simulink model "GIL11_free_mechanism"  (R2019b)
settings: Solver=VariableStepAuto  StartTime=0.133  StopTime=1.0823  MaxStep=0.01  RelTol=1e-3
PreLoadFcn:
  | kinData_max = 0;
  | kinData_min = 0;
libraries: simulink x3
settings Model: Creator=admin-local  LastModifiedBy=admin-local

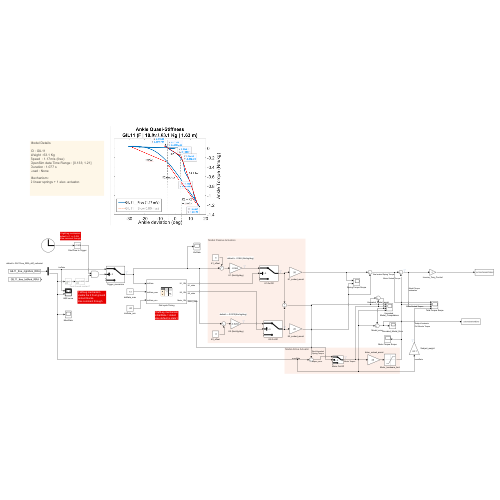
[thumbnail: Simulink's stored preview of the top-level diagram]
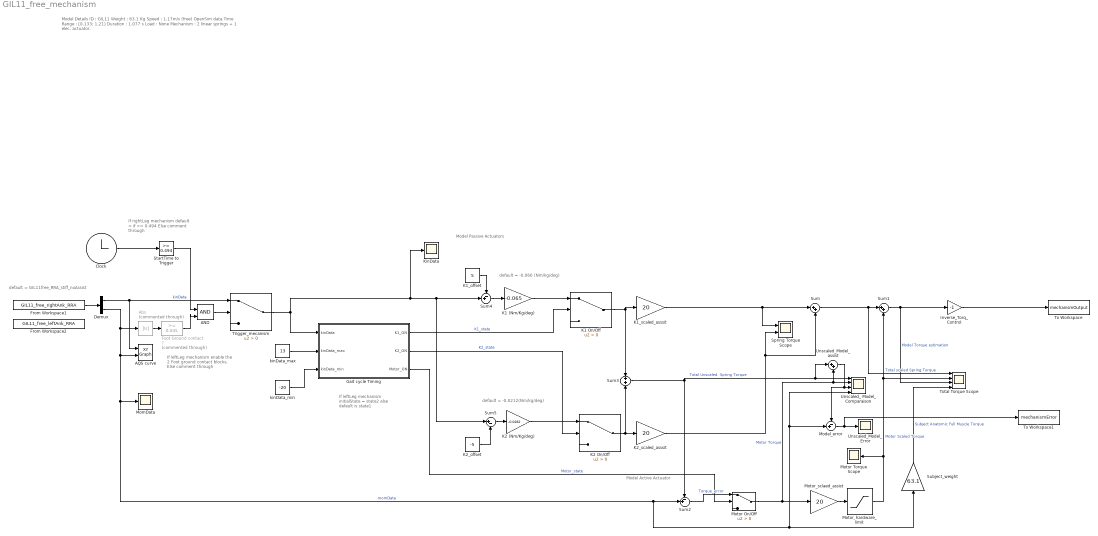
== system GIL11_free_mechanism ==
  note: Model Passive Actuators
  note: default = -0.066 (Nm/kg/deg)
  note: default = -0.0212(Nm/kg/deg)
  note: Model Active Actuator
  note: default = GIL11free_RRA_stiff_noAssist
  note: Model Details
      |
      | ID : GIL11
      | Weight : 63.1 Kg
      | Speed  : 1.17m/s (free)
      | OpenSim data Time Range : [0.133; 1.21]
      | Duration : 1.077 s
      | Load : None
      |
      | Mechanism :
      | 2 linear springs + 1 elec. actuator.
  note: If leftLeg mechanism
      | initialState = state2
      | else default is state1
  note: If rightLeg mechanism
      | default = if  >= 0.494
      | Else comment through
  note: If leftLeg mechanism
      | enable the 2 Foot ground contact blocks.
      | Else comment through
  AND : Logic  IconShape=distinctive  AllPortsSameDT=off  OutDataTypeStr=boolean
  AQS curve : simulink/Sinks/XY Graph  xmin=-1  xmax=1  ymin=-1  ymax=1  st=-1
  Abs : Abs  Commented=through
  Clock : Clock
  Demux : Demux  Outputs=2
  Foot Ground contact ? : simulink/Logic and Bit Operations/Compare To Constant  Commented=through  relop=>=  const=0.045  OutDataTypeStr=boolean
  From Workspace1 : FromWorkspace  VariableName=GIL11_free_rightAnk_RRA  OutputAfterFinalValue=Holding final value
  From Workspace2 : FromWorkspace  VariableName=GIL11_free_leftAnk_RRA  OutputAfterFinalValue=Holding final value
  Gait cycle Timing : State Transition Table  TreatAsAtomicUnit=on
  Inverse_Torq_Control : Gain  Gain=-1
  K1 (Nm/Kg/deg) : Gain  Gain=-0.065
  K1 On/Off : Switch  Criteria=u2 > Threshold
  "K1_offset " : Constant  Value=5
  K1_scaled_asssit : Gain  Gain=20
  K2 (Nm/Kg/deg) : Gain  Gain=-0.0282
  K2 On/Off : Switch  Criteria=u2 > Threshold
  K2_offset : Constant  Value=-5
  K2_scaled_asssit : Gain  Gain=20
  KinData : Scope
  Model_error : Sum  Inputs=-+|
  "MomData " : Scope
  Motor On/Off : Switch  Criteria=u2 > Threshold
  Motor Torque Scope : Scope
  Motor_hardware_limit : Saturate  UpperLimit=16  LowerLimit=-16
  Motor_sclaed_assist : Gain  Gain=20
  Spring Torque Scope : Scope  NumInputPorts=2
  StartTime to Trigger : simulink/Logic and Bit Operations/Compare To Constant  relop=>=  const=0.494  OutDataTypeStr=boolean
  Subject_weight : Gain  Gain=63.1
  Sum : Sum  Inputs=|++
  Sum1 : Sum  Inputs=|++
  Sum2 : Sum  Inputs=-+|
  Sum3 : Sum  Inputs=+|+
  Sum4 : Sum  Inputs=-+|
  Sum5 : Sum  Inputs=|+-
  To Workspace : ToWorkspace  VariableName=mechanismOutput  SaveFormat=Timeseries  SampleTime=-1
  To Workspace1 : ToWorkspace  VariableName=mechanismError  SaveFormat=Timeseries  SampleTime=-1
  Total Torque Scope : Scope  NumInputPorts=4
  Trigger_mecanism : Switch  Criteria=u2 > Threshold
  Unscaled_ Model_Comparaison : Scope  NumInputPorts=4
  Unscaled_Model_Error : Scope
  Unscaled_Model_assist : Sum  Inputs=|++
  "kinData_max " : Constant  Value=13
  "kinData_min " : Constant  Value=-20
  wires:
  Gait cycle Timing/1(K1_ON) -> K1 On/Off/2  "K1_state"
  Motor On/Off/1 -> Unscaled_Model_assist/2, Unscaled_ Model_Comparaison/2, Motor_sclaed_assist/1  "Motor Torque"
  Gait cycle Timing/2(K2_ON) -> K2 On/Off/2  "K2_state"
  "kinData_max "/1 -> Gait cycle Timing/2(kinData_max)
  Gait cycle Timing/3(Motor_ON) -> Motor On/Off/2  "Motor_state"
  Demux/1 -> Trigger_mecanism/1, AQS curve/1  "kinData"
  Sum2/1 -> Motor On/Off/1  "Torque_error"
  Sum1/1 -> Total Torque Scope/3, Inverse_Torq_Control/1  "Model Torque estimation"
  K1_scaled_asssit/1 -> Spring Torque Scope/1, Sum/1
  "kinData_min "/1 -> Gait cycle Timing/3(kinData_min)
  Demux/2 -> Abs/1, AQS curve/2, "MomData "/1, Subject_weight/1, Model_error/2, Unscaled_ Model_Comparaison/4, Sum2/2  "momData"
  "K1_offset "/1 -> Sum4/1
  K2_offset/1 -> Sum5/2
  K1 On/Off/1 -> K1_scaled_asssit/1, Sum3/1
  Sum4/1 -> K1 (Nm/Kg/deg)/1
  Sum5/1 -> K2 (Nm/Kg/deg)/1
  K2 On/Off/1 -> K2_scaled_asssit/1, Sum3/2
  K1 (Nm/Kg/deg)/1 -> K1 On/Off/1
  K2 (Nm/Kg/deg)/1 -> K2 On/Off/1
  Subject_weight/1 -> Total Torque Scope/4  "Subject Anatomic Full Muscle Torque"
  Inverse_Torq_Control/1 -> To Workspace/1
  Sum3/1 -> Unscaled_Model_assist/1, Unscaled_ Model_Comparaison/1, Sum2/1  "Total Unscaled  Spring Torque"
  K2_scaled_asssit/1 -> Spring Torque Scope/2, Sum/2
  Sum/1 -> Total Torque Scope/1, Sum1/1  "Total scaled Spring Torque"
  Motor_hardware_limit/1 -> Total Torque Scope/2, Sum1/2, Motor Torque Scope/1  "Motor Scaled Torque"
  Motor_sclaed_assist/1 -> Motor_hardware_limit/1
  Trigger_mecanism/1 -> Sum4/2, Sum5/1, KinData/1, Gait cycle Timing/1(kinData)
  Unscaled_Model_assist/1 -> Model_error/1, Unscaled_ Model_Comparaison/3
  Clock/1 -> StartTime to Trigger/1
  AND/1 -> Trigger_mecanism/2
  StartTime to Trigger/1 -> AND/1
  Abs/1 -> Foot Ground contact ?/1
  Foot Ground contact ?/1 -> AND/2
  Model_error/1 -> To Workspace1/1, Unscaled_Model_Error/1
  From Workspace1/1 -> Demux/1

== stateflow chart GIL11_free_mechanism/Gait cycle Timing ==
  state state1
    K2_ON = 0
  state state2
    K2_ON = 1
  state state3
  state state4
  state state5
  state state6
  (default) -> state1
  (junction 260) -> state1
  (junction 262) -> (junction 260)
  state1 -> state2 : [kinData <= -5 & K2_ON == 0]
      | {K1_ON= 0;
      | K2_ON = 1;
      | Motor_ON = 0;}
  state2 -> (junction 252) [order 2] : [kinData > -5 & kinData <= 1 ]
      | {K1_ON= 0;
      | K2_ON = 0;
      | Motor_ON = 0;}
  (junction 252) -> state2
  state2 -> state3 [order 1] : [kinData > 5]
      | {K1_ON= 1;
      | K2_ON = 1;
      | Motor_ON = 0;}
  state3 -> state4 : [kinData >= kinData_max]
      | {K1_ON= 1;
      | K2_ON = 1;
      | Motor_ON = 1;}
  state4 -> state5 : [kinData <= 5]
      | {K1_ON= 0;
      | K2_ON = 1;
      | Motor_ON = 1;}
  state5 -> state6 : [kinData <= -5]
      | {K1_ON= 0;
      | K2_ON = 0;
      | Motor_ON = 1;}
  state6 -> (junction 262) : [kinData <= kinData_min]
      | {K1_ON= 0;
      | K2_ON = 0;
      | Motor_ON = 0;}
  data: kinData input; K1_ON output; K2_ON output; Motor_ON output; kinData_max input; kinData_min input
